simulink model "LAB2_Response"  (R2025a)
settings: Solver=VariableStepAuto  StartTime=0.0  StopTime=6.4  RelTol=1e-3
settings Model: Creator=title  LastModifiedBy=title

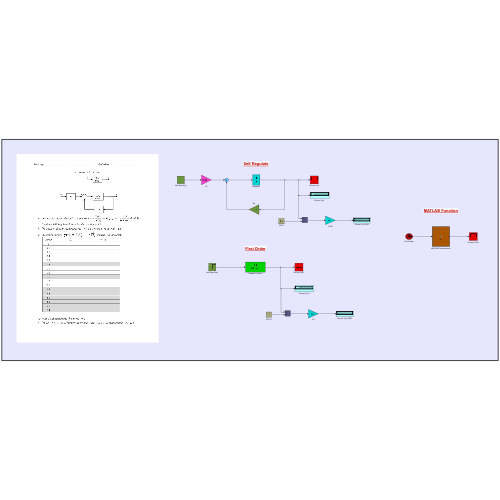
[thumbnail: Simulink's stored preview of the top-level diagram]
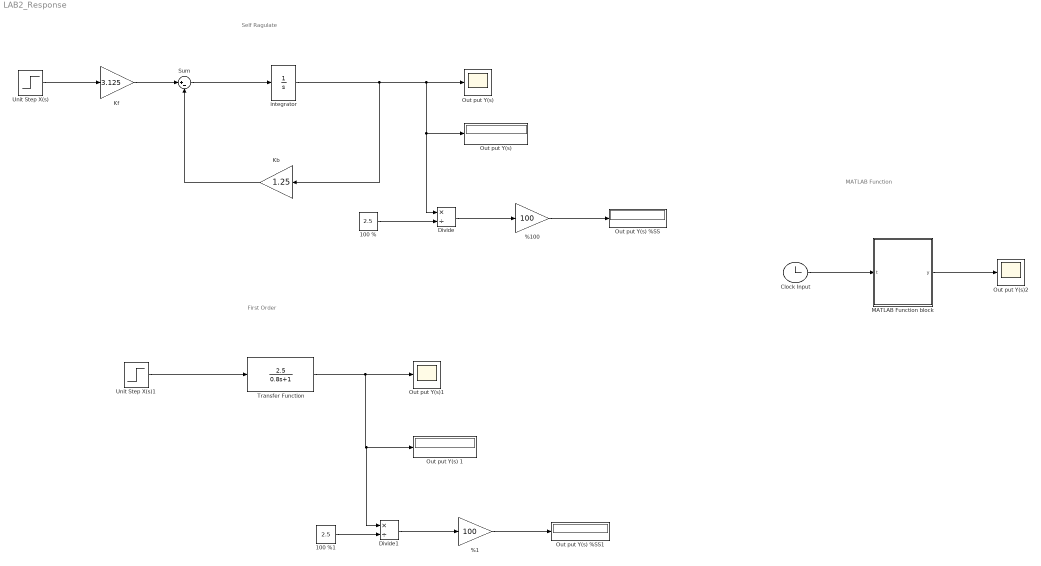
== system LAB2_Response ==
  note: Self Ragulate
  note: First Order
  note: MATLAB Function
  %1 : Gain  Gain=100
  %100 : Gain  Gain=100
  100 % : Constant  Value=2.5
  100 %1 : Constant  Value=2.5
  Clock Input : Clock
  Divide : Product  Inputs=*/
  Divide1 : Product  Inputs=*/
  Kb : Gain  Gain=1.25
  Kf : Gain  Gain=3.125
  MATLAB Function block : MATLAB Function  TreatAsAtomicUnit=on
  Out put Y(s) : Scope
      settings: ActiveDisplayYMinimum=-1  ActiveDisplayYMaximum=1
  "Out put Y(s) " : Display
  Out put Y(s) %SS : Display
  Out put Y(s) %SS1 : Display
  Out put Y(s) 1 : Display
  Out put Y(s)1 : Scope
      settings: ActiveDisplayYMinimum=-1  ActiveDisplayYMaximum=1
  Out put Y(s)2 : Scope
      settings: ActiveDisplayYMinimum=-1  ActiveDisplayYMaximum=1  DataLoggingVariableName=ScopeData2
  Sum : Sum  Inputs=|+-
  Transfer Function : TransferFcn  Numerator=2.5  Denominator=[0.8 1]
  Unit Step X(s) : Step  Time=0  SampleTime=0
  Unit Step X(s)1 : Step  Time=0  SampleTime=0
  integrator : Integrator
  wires:
  Unit Step X(s)/1 -> Kf/1
  Sum/1 -> integrator/1
  Kb/1 -> Sum/2
  Kf/1 -> Sum/1
  integrator/1 -> Kb/1, Out put Y(s)/1, Divide/1, "Out put Y(s) "/1
  100 %/1 -> Divide/2
  Divide/1 -> %100/1
  %100/1 -> Out put Y(s) %SS/1
  Unit Step X(s)1/1 -> Transfer Function/1
  Transfer Function/1 -> Divide1/1, Out put Y(s) 1/1, Out put Y(s)1/1
  Divide1/1 -> %1/1
  %1/1 -> Out put Y(s) %SS1/1
  100 %1/1 -> Divide1/2
  MATLAB Function block/1(y) -> Out put Y(s)2/1
  Clock Input/1 -> MATLAB Function block/1(t)

== matlab function LAB2_Response/MATLAB Function block ==
  data: t input; y output
function y = fcn(t)

y = 2.5*(1-exp(-t/0.8));
end
